simulink model "work6"  (R2026a)
settings: Solver=ode45  StopTime=10  RelTol=1e-8  AbsTol=1e-10
settings Model: Creator=m  LastModifiedBy=m

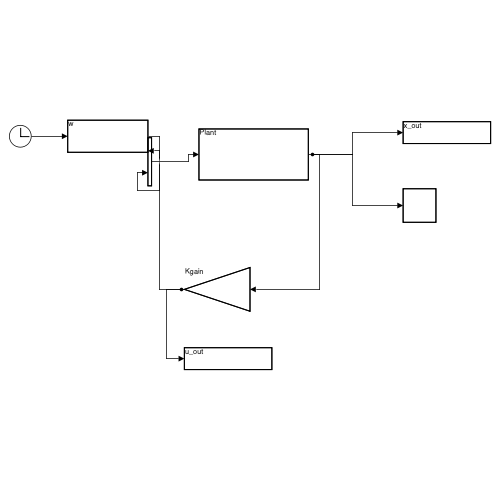
[thumbnail: Simulink's stored preview of the top-level diagram]
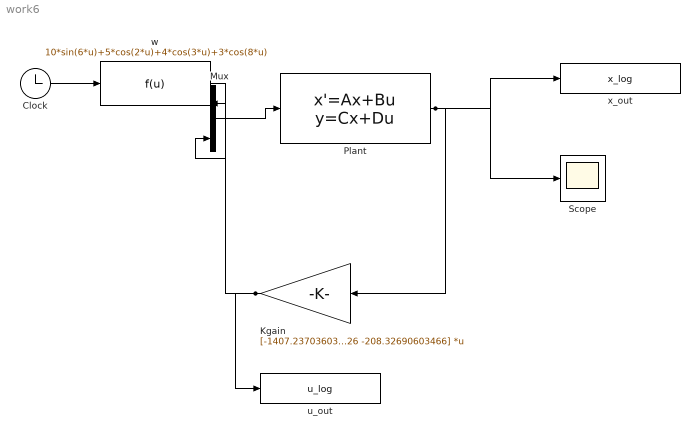
== system work6 ==
  Clock : Clock
  Kgain : Gain  Gain=[-1407.23703603826 -208.32690603466]  Multiplication=Matrix(K*u)
  Mux : Mux  Inputs=2
  Plant : StateSpace  A=[6 2;-3 0]  B=[0 4;3 1]  C=[1 0;0 1]  D=[0 0;0 0]  InitialCondition=[1;0]
  Scope : Scope
  u_out : ToWorkspace  VariableName=u_log  SaveFormat=Timeseries  SampleTime=-1
  w : Fcn  Expr=10*sin(6*u)+5*cos(2*u)+4*cos(3*u)+3*cos(8*u)
  x_out : ToWorkspace  VariableName=x_log  SaveFormat=Timeseries  SampleTime=-1
  wires:
  Plant/1 -> Kgain/1, x_out/1, Scope/1
  Kgain/1 -> Mux/1, u_out/1
  Clock/1 -> w/1
  w/1 -> Mux/2
  Mux/1 -> Plant/1
